simulink model "sensor_fusion"  (R2022b)
settings: Solver=VariableStepAuto  StartTime=0.0  StopTime=5  RelTol=1e-3
values from neighbouring files (symbols this model uses):
  pid_pp_selector = 0    [model_state.mat]    (also in setup_model.m)
  route = [x_xformed' -y_xformed']    [generate_route.m]    (also in model_state.mat = [3.12797877236 3.23666357277 3.40196097956 3.55303789303 3.6; setup_model.m = generate_route(50, 'rand'))
undefined symbols (not defined in the file or in its folder): Angle, Axis
libraries: matrix_library x4, robotcorelib x3, vrlib x3, mspfiltlib x1, robotmobilelib x1, mspsensorlib x1, robotalgslib x1, slpidlib x1
settings Model: Creator=sjohnson  LastModifiedBy=sjohnson

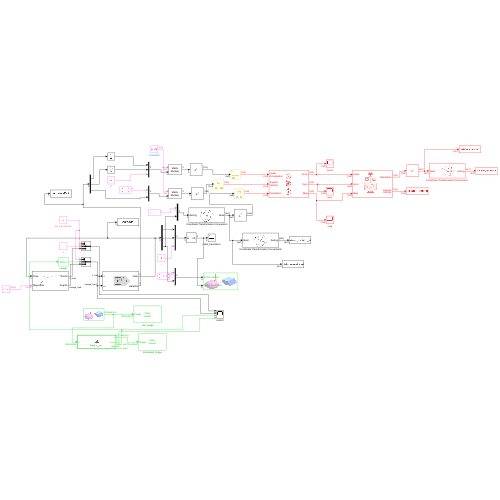
[thumbnail: Simulink's stored preview of the top-level diagram]
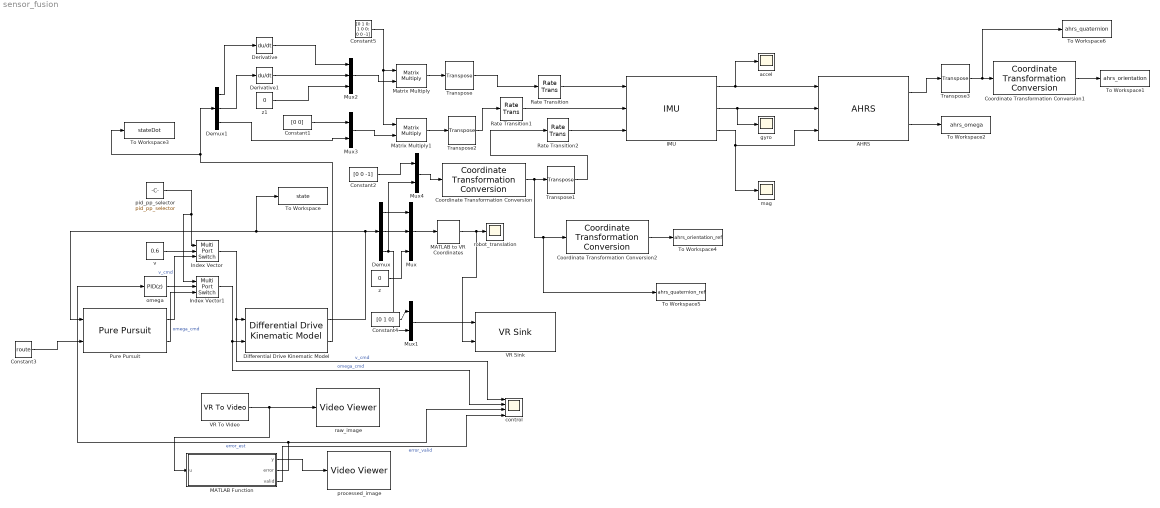
== system sensor_fusion ==
  AHRS : mspfiltlib/AHRS  DispRefFrame=NED  DecimationFactor=1  InitialProcessNoise=ahrsfilter.defaultProcessNoise  OrientationFormat=quaternion  SimulateUsing=Interpreted execution  AccelerometerNoise=0.0001924722  GyroscopeNoise=9.1385e-5  MagnetometerNoise=0.1  GyroscopeDriftNoise=3.0462e-13  LinearAccelerationNoise=0.0096236100000000012  MagneticDisturbanceNoise=0.5  LinearAccelerationDecayFactor=0.5  MagneticDisturbanceDecayFactor=0.5  ExpectedMagneticFieldStrength=50
  Constant1 : Constant  Value=[0 0]
  Constant2 : Constant  Value=[0 0 -1]
  Constant3 : Constant  Value=route
  Constant4 : Constant  Value=[0 1 0]
  Constant5 : Constant  Value=[0 1 0; 1 0 0; 0 0 -1]
  Coordinate Transformation Conversion : robotcorelib/Coordinate Transformation Conversion  InputRepresentation=Axis-Angle  InputEulerSequence=ZYX  ShowTrVecInputPort=on  OutputRepresentation=Quaternion  OutputEulerSequence=ZYX  ShowTrVecOutputPort=on  SimulateUsing=Interpreted execution
  Coordinate Transformation Conversion1 : robotcorelib/Coordinate Transformation Conversion  InputRepresentation=Quaternion  InputEulerSequence=ZYX  ShowTrVecInputPort=on  OutputRepresentation=Axis-Angle  OutputEulerSequence=ZYX  ShowTrVecOutputPort=on  SimulateUsing=Interpreted execution
  Coordinate Transformation Conversion2 : robotcorelib/Coordinate Transformation Conversion  InputRepresentation=Quaternion  InputEulerSequence=ZYX  ShowTrVecInputPort=on  OutputRepresentation=Axis-Angle  OutputEulerSequence=ZYX  ShowTrVecOutputPort=on  SimulateUsing=Interpreted execution
  Demux : Demux  Outputs=3
  Demux1 : Demux  Outputs=3
  Derivative : Derivative  CoefficientInTFapproximation=100
  Derivative1 : Derivative  CoefficientInTFapproximation=100
  Differential Drive Kinematic Model : robotmobilelib/Differential Drive Kinematic Model  VehicleInputs=Vehicle Speed & Heading Angular Velocity  WheelRadius=0.025  WheelSpeedRange=[-inf inf]  TrackWidth=0.1  InitialState=vehicle_initial_state  SimulateUsing=Interpreted execution
  IMU : mspsensorlib/IMU  DispRefFrame=NED  Temperature=20  MagneticFieldNED=[ 27.5550, -2.4169, -16.0849 ]  MagneticFieldENU=[ -2.4169, 27.5550, 16.0849 ]  SeedDouble=67  SimulateUsing=Interpreted execution  AccelParamsMeasurementRange=Inf  AccelParamsResolution=0  AccelParamsConstantBias=[ 0, 0, 0 ]  AccelParamsAxesMisalignment=[ 100, 0, 0; 0, 100, 0; 0, 0, 100 ]  AccelParamsNoiseDensity=[ 0, 0, 0 ]  AccelParamsBiasInstability=[ 0, 0, 0 ]  AccelParamsRandomWalk=[ 0, 0, 0 ]  AccelParamsTemperatureBias=[ 0, 0, 0 ]  AccelParamsTemperatureScaleFactor=[ 0, 0, 0 ]  GyroParamsMeasurementRange=Inf  GyroParamsResolution=0  GyroParamsConstantBias=[ 0, 0, 0 ]  GyroParamsAxesMisalignment=[ 100, 0, 0; 0, 100, 0; 0, 0, 100 ]  GyroParamsAccelerationBias=[ 0, 0, 0 ]  GyroParamsNoiseDensity=[ 0, 0, 0 ]  GyroParamsBiasInstability=[ 0, 0, 0 ]  GyroParamsRandomWalk=[ 0, 0, 0 ]  GyroParamsTemperatureBias=[ 0, 0, 0 ]  GyroParamsTemperatureScaleFactor=[ 0, 0, 0 ]  MagParamsMeasurementRange=Inf  MagParamsResolution=0  MagParamsConstantBias=[ 0, 0, 0 ]  MagParamsAxesMisalignment=[ 100, 0, 0; 0, 100, 0; 0, 0, 100 ]  MagParamsNoiseDensity=[ 0, 0, 0 ]  MagParamsBiasInstability=[ 0, 0, 0 ]  MagParamsRandomWalk=[ 0, 0, 0 ]  MagParamsTemperatureBias=[ 0, 0, 0 ]  MagParamsTemperatureScaleFactor=[ 0, 0, 0 ]
  Index Vector : MultiPortSwitch  DataPortOrder=Zero-based contiguous  Inputs=2  zeroidx=on  SaturateOnIntegerOverflow=off  InputSameDT=off
  Index Vector1 : MultiPortSwitch  DataPortOrder=Zero-based contiguous  Inputs=2  zeroidx=on  SaturateOnIntegerOverflow=off  InputSameDT=off
  MATLAB Function : MATLAB Function  TreatAsAtomicUnit=on
  MATLAB to VR Coordinates : vrlib/Utilities/MATLAB to VR Coordinates
  Matrix Multiply : Product  Multiplication=Matrix(*)
  Matrix Multiply1 : Product  Multiplication=Matrix(*)
  Mux : Mux  Inputs=3
  Mux1 : Mux  Inputs=2
  Mux2 : Mux  Inputs=3
  Mux3 : Mux  Inputs=2
  Mux4 : Mux  Inputs=2
  Pure Pursuit : robotalgslib/Pure Pursuit  DesiredLinearVelocity=0.75  MaxAngularVelocity=1  LookaheadDistance=0.5  TargetDirPort=off  SimulateUsing=Interpreted execution
      settings: LibrarySourceBlock=robotmobilelib/Pure Pursuit
  Rate Transition : RateTransition  OutPortSampleTime=0.01
  Rate Transition1 : RateTransition  OutPortSampleTime=0.01
  Rate Transition2 : RateTransition  OutPortSampleTime=0.01
  To Workspace : ToWorkspace  VariableName=state  SaveFormat=Structure With Time  SampleTime=-1
  To Workspace1 : ToWorkspace  VariableName=ahrs_orientation  SaveFormat=Structure With Time  SampleTime=-1
  To Workspace2 : ToWorkspace  VariableName=ahrs_omega  SaveFormat=Structure With Time  SampleTime=-1
  To Workspace3 : ToWorkspace  VariableName=stateDot  SaveFormat=Structure With Time  SampleTime=-1
  To Workspace4 : ToWorkspace  VariableName=ahrs_orientation_ref  SaveFormat=Structure With Time  SampleTime=-1
  To Workspace5 : ToWorkspace  VariableName=ahrs_quaternion_ref  SaveFormat=Structure With Time  SampleTime=-1
  To Workspace6 : ToWorkspace  VariableName=ahrs_quaternion  SaveFormat=Structure With Time  SampleTime=-1
  Transpose{,1..3} (4 alike) : matrix_library/Transpose
  VR Sink : vrlib/VR Sink  InstantiateOnLoad=on  SampleTime=0.02  ViewEnable=on  RemoteChange=off  RemoteView=off  FieldsWritten=Robot.rotation.4.1.1.double#Robot.translation.3.1.1.double  WorldFileName=vr_route.x3d  WorldDescription=Differential Wheeled Robot in a Maze  AutoView=on  VideoDimensions=[]  AllowVariableSize=off  FigureProperties="{'Position', 'Name', 'Viewpoint', 'CameraBound', 'CameraDirection', 'CameraPosition', 'CameraUpVector', 'ZoomFactor', 'Antialiasing', 'Headlight', 'Lighting', 'NavPanel', 'Sound', 'StatusBar', 'Stereo3D', 'Stereo3DCameraOffset', 'Stereo3DHIT', 'ToolBar', 'Textures', 'Transparency', 'Triad', 'Wireframe', 'NavZones', 'NavMode', 'NavSpeed', 'CaptureFileFormat', 'CaptureFileName', 'Record2DCompressMethod', 'Record2DCompressQuality', 'Record2D', 'Record2DFileName', 'Record2DFPS'; [9.2500000000000000e+02   1.2900000000000000e+02   5.7600000000000000e+02   3.5000000000000000e+02], 'Differential Wheeled Robot in a Maze', 'Overview', 'on', [0.0000000000000000e+00   0.0000000000000000e+00  -1.0000000000000000e+00], [0.0000000000000000e+00   0.0000000000000000e+00   0.0000000000000000e+00], [0.0000000000000000e+00   1.0000000000000000e+00   0.0000000000000000e+00], [1.0000000000000000e+00], 'on', 'on', 'on', 'halfbar', 'on', 'on', 'off', [1.0000000149011612e-01], [0.0000000000000000e+00], 'on', 'on', 'on', 'none', 'off', 'off', 'fly', 'normal', 'tif', '%f_anim_%n.tif', 'auto', [7.5000000000000000e+01], 'off', '%f_anim_%n.avi', 'auto'}"
  VR To Video : vrlib/VR To Video  InstantiateOnLoad=on  SampleTime=0.02  ViewEnable=on  RemoteChange=off  RemoteView=off  WorldFileName=vr_route.x3d  WorldDescription=Differential Wheeled Robot in a Maze  AutoView=off  VideoDimensions=[480 640]  AllowVariableSize=off  FigureProperties="{'Position', 'Name', 'Viewpoint', 'CameraBound', 'CameraDirection', 'CameraPosition', 'CameraUpVector', 'ZoomFactor', 'Antialiasing', 'Headlight', 'Lighting', 'NavPanel', 'Sound', 'StatusBar', 'Stereo3D', 'Stereo3DCameraOffset', 'Stereo3DHIT', 'ToolBar', 'Textures', 'Transparency', 'Triad', 'Wireframe', 'NavZones', 'NavMode', 'NavSpeed', 'CaptureFileFormat', 'CaptureFileName', 'Record2DCompressMethod', 'Record2DCompressQuality', 'Record2D', 'Record2DFileName', 'Record2DFPS'; [9.9000000000000000e+01   9.8000000000000000e+01   5.7600000000000000e+02   3.5000000000000000e+02], 'Differential Wheeled Robot in a Maze', 'Overview', 'on', [0.0000000000000000e+00   0.0000000000000000e+00  -1.0000000000000000e+00], [0.0000000000000000e+00   0.0000000000000000e+00   0.0000000000000000e+00], [0.0000000000000000e+00   1.0000000000000000e+00   0.0000000000000000e+00], [1.0000000000000000e+00], 'on', 'on', 'on', 'halfbar', 'on', 'on', 'off', [1.0000000149011612e-01], [0.0000000000000000e+00], 'on', 'on', 'on', 'none', 'off', 'off', 'fly', 'normal', 'tif', '%f_anim_%n.tif', 'auto', [7.5000000000000000e+01], 'off', '%f_anim_%n.avi', 'auto'; [7.6700000000000000e+02   9.4000000000000000e+01   6.4000000000000000e+02   4.8000000000000000e+02], 'Differential Wheeled Robot in a Maze', 'Follow Robot', 'on', [0.0000000000000000e+00   0.0000000000000000e+00  -1.0000000000000000e+00], [0.0000000000000000e+00   0.0000000000000000e+00   0.0000000000000000e+00], [0.0000000000000000e+00   1.0000000000000000e+00   0.0000000000000000e+00], [1.0000000000000000e+00], 'on', 'on', 'on', 'none', 'on', 'off', 'off', [1.0000000149011612e-01], [0.0000000000000000e+00], 'off', 'on', 'on', 'none', 'off', 'off', 'fly', 'normal', 'tif', '%f_anim_%n.tif', 'auto', [7.5000000000000000e+01], 'off', '***video***', 'auto'}"
  accel : Scope
  control : Scope  NumInputPorts=4
  gyro : Scope
  mag : Scope
  omega : slpidlib/PID Controller  Controller=PID  Form=Parallel  TimeDomain=Discrete-time  UseExternalTs=off  SampleTime=-1  IntegratorMethod=Forward Euler  FilterMethod=Forward Euler  ControllerParametersSource=internal  P=-3  I=0  UseKiTs=off  D=0  N=100  UseFilter=on  TunerSelectOption=Transfer Function Based (PID Tuner App)  InitialConditionSource=internal  InitialConditionForIntegrator=0  InitialConditionForFilter=0  DifferentiatorICPrevScaledInput=0  ExternalReset=none  TrackingMode=off  Kt=1  LimitOutput=off  SatLimitsSource=internal  UpperSaturationLimit=inf  LowerSaturationLimit=-inf  LinearizeAsGain=off  AntiWindupMode=none  Kb=1  LimitIntegrator=off  UpperIntegratorSaturationLimit=inf  LowerIntegratorSaturationLimit=-inf  POutMin=[]  POutMax=[]  IOutMin=[]  IOutMax=[]  DOutMin=[]  DOutMax=[]  NOutMin=[]  NOutMax=[]  SumOutMin=[]  SumOutMax=[]  SaturationOutMin=[]  SaturationOutMax=[]  PParamMin=[]  PParamMax=[]  IParamMin=[]  IParamMax=[]  DParamMin=[]  DParamMax=[]  NParamMin=[]  NParamMax=[]  KbParamMin=[]  KbParamMax=[]  KtParamMin=[]  KtParamMax=[]  KbOutMin=[]  KbOutMax=[]  KtOutMin=[]  KtOutMax=[]  IntegratorOutMin=[]  IntegratorOutMax=[]  FilterOutMin=[]  FilterOutMax=[]  SumI1OutMin=[]  SumI1OutMax=[]  SumI2OutMin=[]  SumI2OutMax=[]  SumI3OutMin=[]  SumI3OutMax=[]  SumI4OutMin=[]  SumI4OutMax=[]  SumDOutMin=[]  SumDOutMax=[]  DifferentiatorOutMin=[]  DifferentiatorOutMax=[]  FilterDiffOutCoefMin=[]  FilterDiffOutCoefMax=[]  ReciprocalOutMin=[]  ReciprocalOutMax=[]  SumDenOutMin=[]  SumDenOutMax=[]  SumNumOutMin=[]  SumNumOutMax=[]  DivideOutMin=[]  DivideOutMax=[]  UdiffTsProdOutMin=[]  UdiffTsProdOutMax=[]  NTsProdOutMin=[]  NTsProdOutMax=[]  UintegralTsProdOutMin=[]  UintegralTsProdOutMax=[]  UngainTsProdOutMin=[]  UngainTsProdOutMax=[]  ClampingZeroOutDataTypeStr=Inherit: Inherit via back propagation  ClampingZeroOutMin=[]  ClampingZeroOutMax=[]  FilterDenConstantOutDataTypeStr=Inherit: Inherit via back propagation  FilterDenConstantOutMin=[]  FilterDenConstantOutMax=[]  PCopyOutDataTypeStr=Inherit: Inherit via back propagation  PCopyOutMin=[]  PCopyOutMax=[]  NCopyOutDataTypeStr=Inherit: Inherit via back propagation  NCopyOutMin=[]  NCopyOutMax=[]  IntegratorContinuousStateAttributes=''  IntegratorStateMustResolveToSignalObject=off  IntegratorRTWStateStorageClass=Auto  FilterContinuousStateAttributes=''  FilterStateMustResolveToSignalObject=off  FilterRTWStateStorageClass=Auto  ParallelPVariant=InternalParameters  IdealPVariant=Disabled  IVariant=InternalParameters  DVariant=InternalParameters  IntegratorVariant=Discrete  SatVariant=Disabled  AWVariant=Passthrough  PCopyVariant=Disabled  TRVariant=Disabled  FdbkBlocksVariant=Forward  IdealPFdbkVariant=Disabled  SatFdbkVariant=Disabled  DerivativeFilterVariant=ForwardEulerFilter  NVariant=InternalParameters  NCopyVariant=Disabled  FilterICVariant=InternalICsFilter  IntegratorICVariant=InternalICs  ExternalResetVariant=Disabled  TRSumVariant=Passthrough  SumFdbkVariant=Disabled  SumVariant=Sum_PID  TsampFilterVariant=InternalTs  TsampNgainVariant=Passthrough  TsampIntegralVariant=Passthrough  ExternalSaturationOutDataTypeStr=Inherit: Same as second input
      settings: LibrarySourceBlock=simulink/Discrete/Discrete PID Controller
  pid_pp_selector : Constant  Value=pid_pp_selector
  processed_image : VideoViewer  FigPos=[-1751 323 803 189]
  raw_image : VideoViewer  FigPos=[-1426 781 855 643]
  robot_translation : Scope
  v : Constant  Value=0.6
  z : Constant  Value=0
  z1 : Constant  Value=0  VectorParams1D=off
  wires:
  Demux/3 -> Mux4/2, Mux1/2
  Demux/1 -> Mux/1
  MATLAB Function/2(error) -> omega/1, control/3  "error_est"
  MATLAB to VR Coordinates/1 -> VR Sink/2, robot_translation/1
  Index Vector/1 -> control/1, Differential Drive Kinematic Model/1  "v_cmd"
  VR To Video/1 -> MATLAB Function/1(u), raw_image/1
  Mux1/1 -> VR Sink/1
  Index Vector1/1 -> control/2, Differential Drive Kinematic Model/2  "omega_cmd"
  Mux/1 -> MATLAB to VR Coordinates/1
  Constant3/1 -> Pure Pursuit/2
  Constant4/1 -> Mux1/1
  MATLAB Function/3(valid) -> control/4  "error_valid"
  MATLAB Function/1(y) -> processed_image/1
  omega/1 -> Index Vector1/2
  pid_pp_selector/1 -> Index Vector1/1, Index Vector/1
  Demux/2 -> Mux/2
  z/1 -> Mux/3
  v/1 -> Index Vector/2
  Differential Drive Kinematic Model/2 -> To Workspace3/1, Demux1/1
  Transpose2/1 -> Rate Transition1/1
  Demux1/1 -> Derivative/1
  Derivative/1 -> Mux2/1
  z1/1 -> Mux2/3
  Coordinate Transformation Conversion/1 -> To Workspace5/1, Coordinate Transformation Conversion2/1, Transpose1/1
  IMU/2 -> AHRS/2, gyro/1
  IMU/3 -> AHRS/3, mag/1
  Transpose/1 -> Rate Transition/1
  Mux2/1 -> Matrix Multiply/2
  Transpose1/1 -> Rate Transition2/1
  Constant1/1 -> Mux3/1
  Demux1/3 -> Mux3/2
  Mux3/1 -> Matrix Multiply1/2
  Demux1/2 -> Derivative1/1
  Derivative1/1 -> Mux2/2
  Differential Drive Kinematic Model/1 -> To Workspace/1, Pure Pursuit/1, Demux/1
  Constant2/1 -> Mux4/1
  Mux4/1 -> Coordinate Transformation Conversion/1
  Rate Transition/1 -> IMU/1
  Rate Transition1/1 -> IMU/2
  Rate Transition2/1 -> IMU/3
  Pure Pursuit/1 -> Index Vector/3  "v_cmd"
  Pure Pursuit/2 -> Index Vector1/3  "omega_cmd"
  IMU/1 -> accel/1, AHRS/1
  AHRS/1 -> Transpose3/1
  AHRS/2 -> To Workspace2/1
  Coordinate Transformation Conversion1/1 -> To Workspace1/1
  Transpose3/1 -> To Workspace6/1, Coordinate Transformation Conversion1/1
  Constant5/1 -> Matrix Multiply1/1, Matrix Multiply/1
  Matrix Multiply/1 -> Transpose/1
  Matrix Multiply1/1 -> Transpose2/1
  Coordinate Transformation Conversion2/1 -> To Workspace4/1

== matlab function sensor_fusion/MATLAB Function ==
  data: u input; y output; error output; valid output
function [y, error, valid] = image_strip(u)
% trim out horizontal slice of image
y = u(275:425, :, :);
dy = double(y);
redness = dy(:,:,1)./vecnorm(dy,2,3);
y_reduction = max(redness,[],1);
fmin = find(y_reduction>0.7, 1, 'first');
fmax = find(y_reduction>0.7, 1, 'last');
if isempty(fmin) | isempty(fmax)
    valid = 0;
    error = nan;
else
    valid = 1;
    min_value = [find(y_reduction>0.7, 1, 'first')];
    max_value = [find(y_reduction>0.7, 1, 'last')];
    error = ((max_value(1) + min_value(1))/2 - 320)/320;
end
